simulink model "part2d1"  (R2016a)
settings: Solver=VariableStepAuto  StartTime=0.0  StopTime=10.0  RelTol=1e-3
libraries: powerlib x11, powerlib_meascontrol x1
settings Model: Creator=St  LastModifiedBy=St

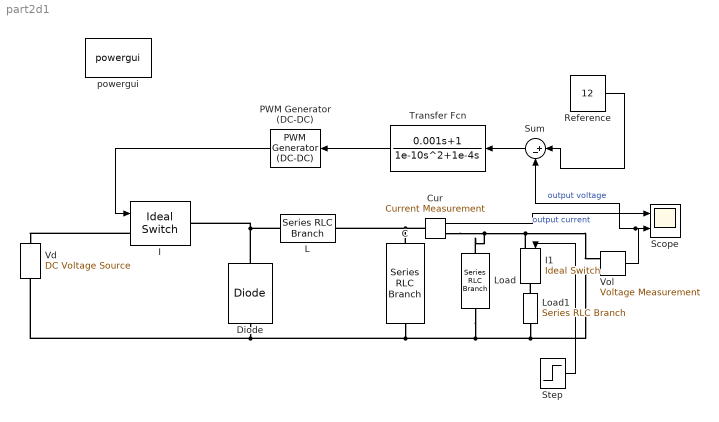
== system part2d1 ==
  C : powerlib/Elements/Series RLC Branch  LConnTagsString=__new0  RConnTagsString=__new0  BranchType=RC  Resistance=0.01  Inductance=1e-3  SetiL0=off  InitialCurrent=0  Capacitance=470e-6  Setx0=off  InitialVoltage=0  Measurements=None
  Cur : powerlib/Measurements/Current Measurement  PhasorSimulation=off  OutputType=Complex  PSBequivalent=0
  Diode : powerlib/Power Electronics/Diode  Ron=0.0000001  Lon=0  Vf=0  IC=0  UseSnubber=off  Rs=inf  Cs=250e-9  Measurements=off
  I : powerlib/Power Electronics/Ideal Switch  Ron=0.00000001  Lon=0  IC=0  Rs=inf  Cs=inf  Measurements=off
  I1 : powerlib/Power Electronics/Ideal Switch  Ron=0.00000001  Lon=0  IC=0  Rs=inf  Cs=inf  Measurements=off
  L : powerlib/Elements/Series RLC Branch  LConnTagsString=__new0  RConnTagsString=__new0  BranchType=RL  Resistance=0.01  Inductance=0.5e-3  SetiL0=off  InitialCurrent=0  Capacitance=1e-6  Setx0=off  InitialVoltage=0  Measurements=None
  Load : powerlib/Elements/Series RLC Branch  LConnTagsString=__new0  RConnTagsString=__new0  BranchType=R  Resistance=18/5  Inductance=1e-3  SetiL0=off  InitialCurrent=0  Capacitance=1e-6  Setx0=off  InitialVoltage=0  Measurements=None
  Load1 : powerlib/Elements/Series RLC Branch  LConnTagsString=__new0  RConnTagsString=__new0  BranchType=R  Resistance=18/5  Inductance=1e-3  SetiL0=off  InitialCurrent=0  Capacitance=1e-6  Setx0=off  InitialVoltage=0  Measurements=None
  PWM Generator (DC-DC) : powerlib_meascontrol/Pulse & Signal Generators/PWM Generator (DC-DC)  Fsw=10000  Ts=0
  Reference : Constant  Value=12
  Scope : Scope  NumInputPorts=2
  Step : Step  Time=3  SampleTime=0
  Sum : Sum  Inputs=|+-
  Transfer Fcn : TransferFcn  Numerator=[0.001 1]  Denominator=[1e-10 1e-4 0]
  Vd : powerlib/Electrical Sources/DC Voltage Source  Amplitude=24  Measurements=None
  Vol : powerlib/Measurements/Voltage Measurement  PhasorSimulation=off  OutputType=Complex  PSBequivalent=0
  powergui : powerlib/powergui  Priority=1  SimulationMode=Continuous  SolverType=Tustin/Backward Euler (TBE)  SampleTime=50e-6  frequency=60  SPID=on  DisableSnubberDevices=off  DisableRonSwitches=off  DisableVfSwitches=off  SwTol=0  DisplayEquations=off  Interpol=off  ExternalGateDelay=off  methode=off  Ts=10  FunctionMessages=off  echomessages=off  HookPort=off  EnableUseOfTLC=off  x0status=blocks  frequencyindice=0  Pbase=100e6  ErrMax=1e-4  Iterations=50  UnitsV=kV  UnitsW=MW  buscounter=0  RestoreLinks=warning  ResistiveCurrentMeasurement=off  Frange=[0:2:500]  Ylog=off  Xlog=on  ShowGrid=off  save=off  variable=ZData  structure=0  ZoomFFT=off  StartTime=0.0  cycles=1  DisplayStyle=1  fundamental=60  FreqAxis=off  MaxFrequency=1000  frequencyindicesteady=1  RmsSteady=1  display=off
  wires:
  Vol/1 -> Sum/2, Scope/2  "output voltage"
  Reference/1 -> Sum/1
  Sum/1 -> Transfer Fcn/1
  Transfer Fcn/1 -> PWM Generator (DC-DC)/1
  PWM Generator (DC-DC)/1 -> I/1
  Cur/1 -> Scope/1  "output current"
  Step/1 -> I1/1
  connections:
  I/LConn1 -- Vd/RConn1
  Diode/RConn1 -- L/LConn1 -- I/RConn1
  Diode/LConn1 -- Vol/LConn2 -- Load1/RConn1 -- Load/RConn1 -- C/RConn1 -- Vd/LConn1
  C/LConn1 -- L/RConn1 -- Cur/LConn1
  Load/LConn1 -- Cur/RConn1 -- Vol/LConn1 -- I1/LConn1
  Load1/LConn1 -- I1/RConn1
